simulink model "zad3_repr_graf_niel_dyn_mod_ciagly_i_dyskretny"  (R2014b)
settings: Solver=ode45  StartTime=0.0  StopTime=70  RelTol=1e-3
values from neighbouring files (symbols this model uses):
  Tp = Tp_vector(k)    [zad_3.m]
undefined symbols (not defined in the file or in its folder): a1, a2, a3, a4, K, T1, T2, x1, x2
settings Model: Creator=Konrad  LastModifiedBy=Konrad

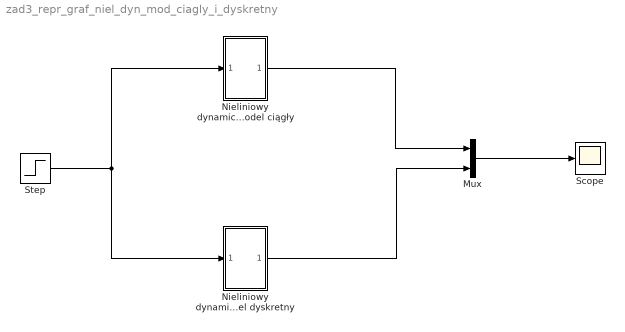
== system zad3_repr_graf_niel_dyn_mod_ciagly_i_dyskretny ==
  Mux : Mux  Inputs=2
  Nieliniowy dynamiczny model ciągły : Subsystem
  Nieliniowy dynamiczny model dyskretny : Subsystem
  Scope : Scope
      settings: YMin=-7  YMax=0
  Step : Step  SampleTime=0
  wires:
  Mux/1 -> Scope/1
  Step/1 -> Nieliniowy dynamiczny model dyskretny/1(u[k]), Nieliniowy dynamiczny model ciągły/1(u(t))
  Nieliniowy dynamiczny model ciągły/1(y(t)) -> Mux/1
  Nieliniowy dynamiczny model dyskretny/1(y[k]) -> Mux/2

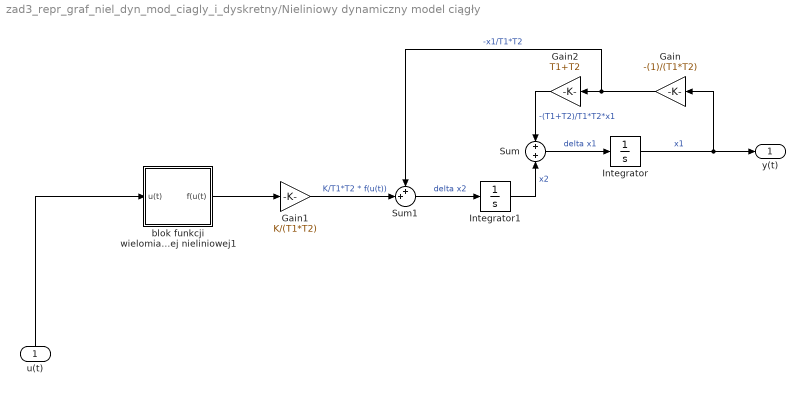
== system zad3_repr_graf_niel_dyn_mod_ciagly_i_dyskretny/Nieliniowy dynamiczny model ciągły ==
  u(t) : Inport
  Gain : Gain  Gain=-(1)/(T1*T2)
  Gain1 : Gain  Gain=K/(T1*T2)
  Gain2 : Gain  Gain=T1+T2
  Integrator : Integrator  InitialCondition=x1  ContinuousStateAttributes='x1'
  Integrator1 : Integrator  InitialCondition=x2  ContinuousStateAttributes='x2'
  Sum : Sum
  Sum1 : Sum  Inputs=++|
  blok funkcji wielomianowej nieliniowej1 : Subsystem
  y(t) : Outport
  wires:
  blok funkcji wielomianowej nieliniowej1/1(f(u(t)) -> Gain1/1
  u(t)/1 -> blok funkcji wielomianowej nieliniowej1/1(u(t))
  Integrator1/1 -> Sum/2  "x2"
  Gain1/1 -> Sum1/2  "K/T1*T2 * f(u(t))"
  Integrator/1 -> y(t)/1, Gain/1  "x1"
  Gain2/1 -> Sum/1  "-(T1+T2)/T1*T2*x1"
  Sum/1 -> Integrator/1  "delta x1"
  Gain/1 -> Sum1/1, Gain2/1  "-x1/T1*T2"
  Sum1/1 -> Integrator1/1  "delta x2"

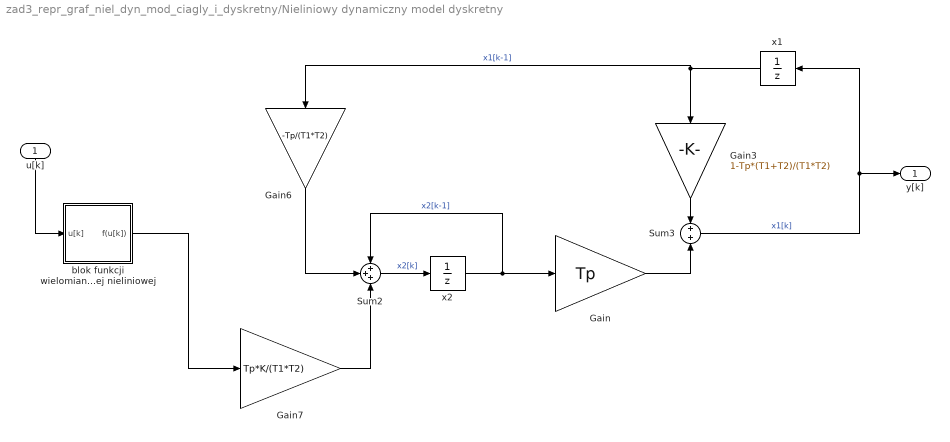
== system zad3_repr_graf_niel_dyn_mod_ciagly_i_dyskretny/Nieliniowy dynamiczny model dyskretny ==
  u[k] : Inport
  Gain : Gain  Gain=Tp
  Gain3 : Gain  Gain=1-Tp*(T1+T2)/(T1*T2)
  Gain6 : Gain  Gain=-Tp/(T1*T2)
  Gain7 : Gain  Gain=Tp*K/(T1*T2)
  Sum2 : Sum  Inputs=+++
  Sum3 : Sum  Inputs=+|+
  blok funkcji wielomianowej nieliniowej : Subsystem
  x1 : UnitDelay  InitialCondition=x1  SampleTime=Tp
  x2 : UnitDelay  InitialCondition=x2  SampleTime=Tp
  y[k] : Outport
  wires:
  u[k]/1 -> blok funkcji wielomianowej nieliniowej/1(u[k])
  Gain7/1 -> Sum2/3
  Gain3/1 -> Sum3/1
  Sum2/1 -> x2/1  "x2[k]"
  Gain/1 -> Sum3/2
  blok funkcji wielomianowej nieliniowej/1(f(u[k])) -> Gain7/1
  Sum3/1 -> x1/1, y[k]/1  "x1[k]"
  x1/1 -> Gain3/1, Gain6/1  "x1[k-1]"
  x2/1 -> Gain/1, Sum2/1  "x2[k-1]"
  Gain6/1 -> Sum2/2

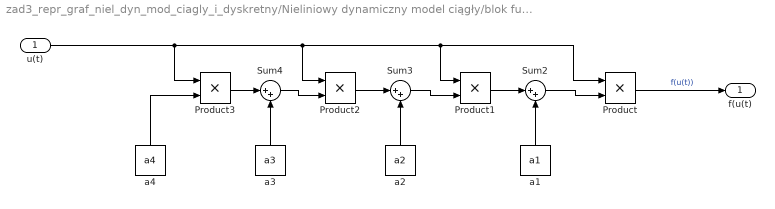
== system zad3_repr_graf_niel_dyn_mod_ciagly_i_dyskretny/Nieliniowy dynamiczny model ciągły/blok funkcji wielomianowej nieliniowej1 ==
  u(t) : Inport
  Product{,1..3} (4 alike) : Product
  Sum2 : Sum  Inputs=|++
  Sum3 : Sum  Inputs=|++
  Sum4 : Sum  Inputs=|++
  a1 : Constant  Value=a1
  a2 : Constant  Value=a2
  a3 : Constant  Value=a3
  a4 : Constant  Value=a4
  f(u(t) : Outport
  wires:
  u(t)/1 -> Product/1, Product1/1, Product2/1, Product3/1
  Product1/1 -> Sum2/1
  Product2/1 -> Sum3/1
  Sum2/1 -> Product/2
  Product/1 -> f(u(t)/1  "f(u(t))"
  Product3/1 -> Sum4/1
  a1/1 -> Sum2/2
  a2/1 -> Sum3/2
  Sum3/1 -> Product1/2
  a3/1 -> Sum4/2
  Sum4/1 -> Product2/2
  a4/1 -> Product3/2

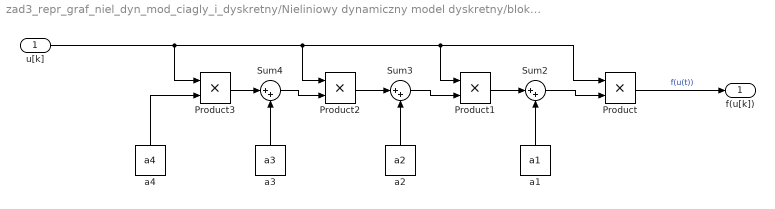
== system zad3_repr_graf_niel_dyn_mod_ciagly_i_dyskretny/Nieliniowy dynamiczny model dyskretny/blok funkcji wielomianowej nieliniowej ==
  u[k] : Inport
  Product{,1..3} (4 alike) : Product
  Sum2 : Sum  Inputs=|++
  Sum3 : Sum  Inputs=|++
  Sum4 : Sum  Inputs=|++
  a1 : Constant  Value=a1
  a2 : Constant  Value=a2
  a3 : Constant  Value=a3
  a4 : Constant  Value=a4
  f(u[k]) : Outport
  wires:
  u[k]/1 -> Product/1, Product1/1, Product2/1, Product3/1
  Product1/1 -> Sum2/1
  Product2/1 -> Sum3/1
  Sum2/1 -> Product/2
  Product/1 -> f(u[k])/1  "f(u(t))"
  Product3/1 -> Sum4/1
  a1/1 -> Sum2/2
  a2/1 -> Sum3/2
  Sum3/1 -> Product1/2
  a3/1 -> Sum4/2
  Sum4/1 -> Product2/2
  a4/1 -> Product3/2
